simulink model "simulation"  (R2022b)
settings: Solver=VariableStepAuto  StartTime=0.0  StopTime=10.0  RelTol=1e-3
values from neighbouring files (symbols this model uses):
  p1 = 0.0002    [bergman.m]    (also in model.m = -0.021151)
  p3 = 0.0001    [bergman.m]    (also in model.m = -0.014188)
  p4 = 0.077947    [model.m]
undefined symbols (not defined in the file or in its folder): d
settings Model: Creator=mhast  LastModifiedBy=mhast

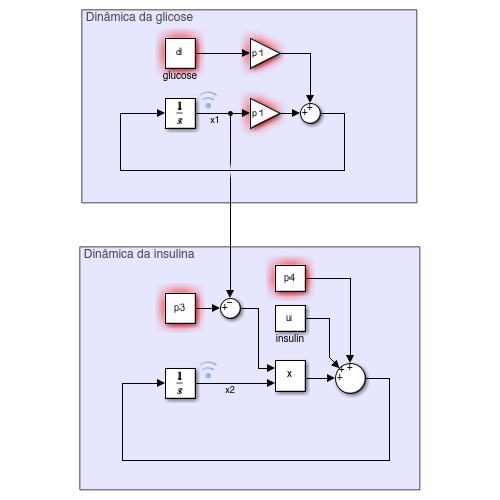
[thumbnail: Simulink's stored preview of the top-level diagram]
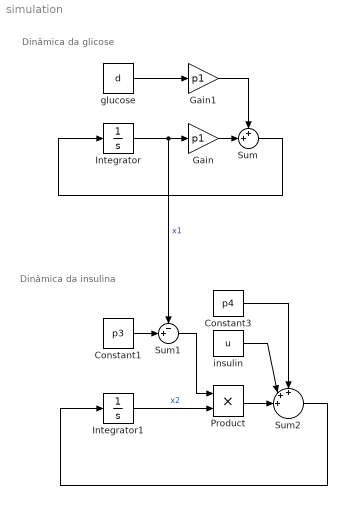
== system simulation ==
  note: Dinâmica da glicose
  note: Dinâmica da insulina
  Constant1 : Constant  Value=p3
  Constant3 : Constant  Value=p4
  Gain : Gain  Gain=p1
  Gain1 : Gain  Gain=p1
  Integrator : Integrator
  Integrator1 : Integrator
  Product : Product
  Sum : Sum  Inputs=++|
  Sum1 : Sum  Inputs=-+|
  Sum2 : Sum  Inputs=+++||
  glucose : Constant  Value=d
  insulin : Constant  Value=u
  wires:
  Sum/1 -> Integrator/1
  Integrator/1 -> Sum1/1, Gain/1  "x1"
  Gain/1 -> Sum/2
  Gain1/1 -> Sum/1
  glucose/1 -> Gain1/1
  Constant1/1 -> Sum1/2
  Sum1/1 -> Product/1
  Integrator1/1 -> Product/2  "x2"
  Product/1 -> Sum2/3
  Constant3/1 -> Sum2/1
  insulin/1 -> Sum2/2
  Sum2/1 -> Integrator1/1
